simulink model "fz8_7"  (R2014a)
settings: Solver=ode45  StartTime=0.0  StopTime=1  RelTol=1e-3
values from neighbouring files (symbols this model uses):
  BER = ber(ii)    [eg8_7.m]    (also in eg8_9.m)
undefined symbols (not defined in the file or in its folder): rsgenpoly
libraries: commblkcod2 x2, commchan3 x1, commsink2 x1, commrandsrc2 x1
settings Model: Creator=tzb  LastModifiedBy=tzb
settings DebuggingCC: SolverPrmCheckMsg=none

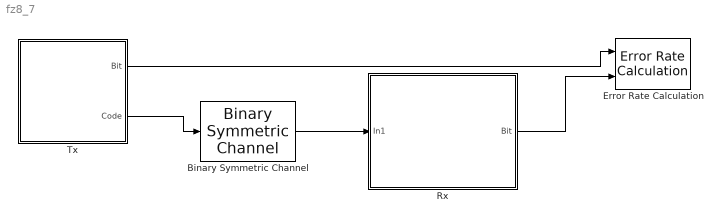
== system fz8_7 ==
  Binary Symmetric Channel : commchan3/Binary Symmetric Channel  P=BER  s=71  E=off  outDtype=double
  Error Rate Calculation : commsink2/Error Rate Calculation  N=0  st_delay=0  cp_mode=Entire frame  subframe=[]  PMode=Workspace  WsName=BER1  RsMode2=off  stop=off  numErr=100  maxBits=1e6
  Rx : Subsystem
  Tx : Subsystem
  wires:
  Rx/1(Bit) -> Error Rate Calculation/2
  Tx/1(Bit) -> Error Rate Calculation/1
  Tx/2(Code) -> Binary Symmetric Channel/1
  Binary Symmetric Channel/1 -> Rx/1(In1)

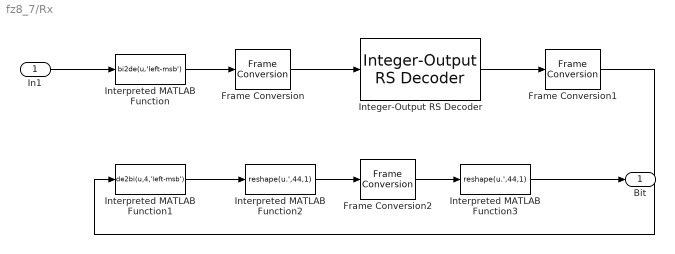
== system fz8_7/Rx ==
  In1 : Inport
  Frame Conversion : FrameConversion
  Frame Conversion1 : FrameConversion  OutFrame=Sample-based
  Frame Conversion2 : FrameConversion
  Integer-Output RS Decoder : commblkcod2/Integer-Output RS Decoder  n=15  k=11  specPrimPoly=off  prPoly=[1 0 1 1]  specGenPoly=off  genPoly=rsgenpoly(7,3)  specPuncture=off  punctVec=[ones(2,1); zeros(2,1)]  specErasurePort=off  showNumErr=off
  Interpreted MATLAB Function : MATLABFcn  MATLABFcn=bi2de(u,'left-msb')
  Interpreted MATLAB Function1 : MATLABFcn  MATLABFcn=de2bi(u,4,'left-msb')  Output1D=off
  Interpreted MATLAB Function2 : MATLABFcn  MATLABFcn=reshape(u.',44,1)  Output1D=off
  Interpreted MATLAB Function3 : MATLABFcn  MATLABFcn=reshape(u.',44,1)  OutputSignalType=real  Output1D=off
  Bit : Outport
  wires:
  Interpreted MATLAB Function2/1 -> Frame Conversion2/1
  Integer-Output RS Decoder/1 -> Frame Conversion1/1
  Frame Conversion2/1 -> Interpreted MATLAB Function3/1
  In1/1 -> Interpreted MATLAB Function/1
  Interpreted MATLAB Function/1 -> Frame Conversion/1
  Frame Conversion/1 -> Integer-Output RS Decoder/1
  Frame Conversion1/1 -> Interpreted MATLAB Function1/1
  Interpreted MATLAB Function1/1 -> Interpreted MATLAB Function2/1
  Interpreted MATLAB Function3/1 -> Bit/1

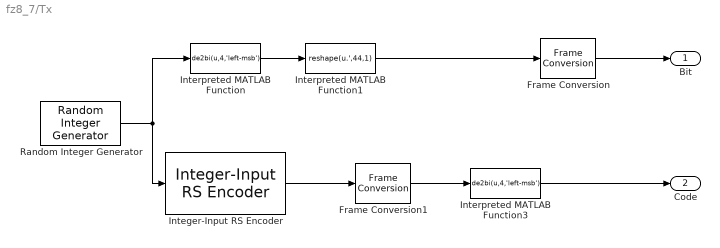
== system fz8_7/Tx ==
  Frame Conversion : FrameConversion
  Frame Conversion1 : FrameConversion  OutFrame=Sample-based
  Integer-Input RS Encoder : commblkcod2/Integer-Input RS Encoder  n=15  k=11  specPrimPoly=off  prPoly=[1 0 1 1]  specGenPoly=off  genPoly=rsgenpoly(7,3)  specPuncture=off  punctVec=[ones(2,1); zeros(2,1)]
  Interpreted MATLAB Function : MATLABFcn  MATLABFcn=de2bi(u,4,'left-msb')  Output1D=off
  Interpreted MATLAB Function1 : MATLABFcn  MATLABFcn=reshape(u.',44,1)  OutputSignalType=real  Output1D=off
  Interpreted MATLAB Function3 : MATLABFcn  MATLABFcn=de2bi(u,4,'left-msb')  Output1D=off
  Random Integer Generator : commrandsrc2/Random Integer Generator  mul=16  seed=37  Ts=1/110000  frameBased=on  sampPerFrame=11  orient=off  outDataType=double
  Bit : Outport
  Code : Outport  Port=2
  wires:
  Random Integer Generator/1 -> Interpreted MATLAB Function/1, Integer-Input RS Encoder/1
  Interpreted MATLAB Function3/1 -> Code/1
  Frame Conversion1/1 -> Interpreted MATLAB Function3/1
  Frame Conversion/1 -> Bit/1
  Integer-Input RS Encoder/1 -> Frame Conversion1/1
  Interpreted MATLAB Function/1 -> Interpreted MATLAB Function1/1
  Interpreted MATLAB Function1/1 -> Frame Conversion/1
